simulink subsystem "Modelo_Sensores"  (R2023b)
settings: Solver=VariableStepAuto  StartTime=0.0  StopTime=10.0  RelTol=1e-3
libraries: arduinolib x2
settings Model: Creator=pablo  LastModifiedBy=pablo

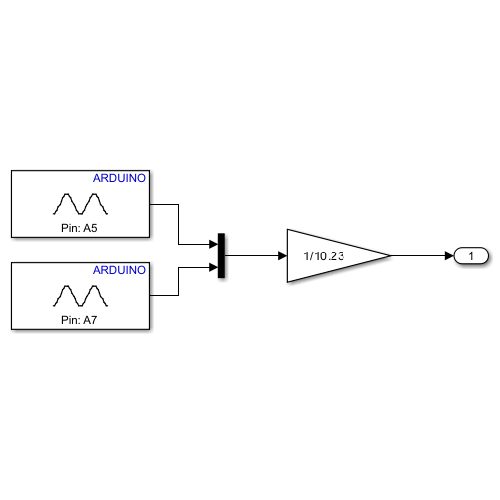
[thumbnail: Simulink's stored preview of the top-level diagram]
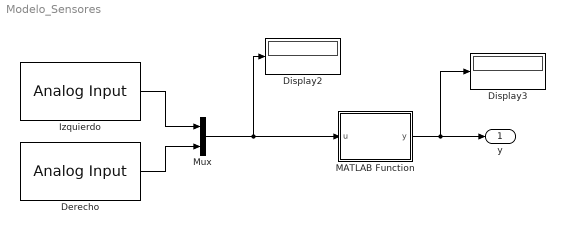
== system Modelo_Sensores ==
  Derecho : arduinolib/Analog Input  pinNumber=8  ReadResultsOnly=off  ConversionTriggerSource=Software  ExternalTriggerType=uint32( 0 )  OutputDataType=uint16  EnableConversionCompleteNotify=off  EnableOuputStatus=off  SampleTime=0.1  blockPlatform=arduino
  Display2 : Display
  Display3 : Display
  Izquierdo : arduinolib/Analog Input  pinNumber=12  ReadResultsOnly=off  ConversionTriggerSource=Software  ExternalTriggerType=uint32( 0 )  OutputDataType=uint16  EnableConversionCompleteNotify=off  EnableOuputStatus=off  SampleTime=0.1  blockPlatform=arduino
  MATLAB Function : MATLAB Function  TreatAsAtomicUnit=on
  Mux : Mux  Inputs=2
  y : Outport
  wires:
  Izquierdo/1 -> Mux/1
  Derecho/1 -> Mux/2
  Mux/1 -> MATLAB Function/1(u), Display2/1
  MATLAB Function/1(y) -> Display3/1, y/1

== matlab function Modelo_Sensores/MATLAB Function ==
  data: u input; y output
function y = fcn(u)
y = 17569.7*double(u).^(-1.2062);
